simulink model "eFL_control"  (R2025b)
settings: Solver=ode3  StartTime=0.0  StopTime=1.5  FixedStep=1e-5  RelTol=1e-3  EnableMultiTasking=on
values from neighbouring files (symbols this model uses):
  C = 470*10^-6    (= 0.00047)    [plotting.m]    (also in robusnost_grafici.m)
  k0 = 2*200    (= 400)    [plotting.m]    (also in robusnost_grafici.m)
  k1 = 1    [plotting.m]    (also in robusnost_grafici.m)
  ki = 200^2    (= 40000)    [plotting.m]    (also in robusnost_grafici.m)
  L = 15.91*10^-3    (= 0.01591)    [plotting.m]    (also in robusnost_grafici.m = 0.012728)
  poremecaj = 0.8    [plotting.m]    (also in robusnost_grafici.m)
  R = 52    [plotting.m]    (also in robusnost_grafici.m)
  sig2 = (0.02*x2e)^2    (= 0.2025)    [plotting.m]    (also in robusnost_grafici.m = 0)
  x2e = Vc    (= -22.5)    [plotting.m]    (also in robusnost_grafici.m)
settings Model: Creator=Stevica  LastModifiedBy=User
settings SolverCC: AlgebraicLoopSolver=TrustRegion
settings DataIOCC: LimitDataPoints=on  SaveFormat=Array
settings OptimizationCC: LifeSpan=inf
settings DebuggingCC: UnderspecifiedInitializationDetection=Classic  MergeDetectMultiDrivingBlocksExec=none  SolverPrmCheckMsg=warning  UnconnectedInputMsg=warning  UnconnectedOutputMsg=warning  UnconnectedLineMsg=warning  SFUnexpectedBacktrackingDiag=warning  SFNoUnconditionalDefaultTransitionDiag=warning  SFExecutionAtInitializationDiag=none  ArithmeticOperatorsInVariantConditions=warning
settings HardwareCC: ProdBitPerPointer=32.0  ProdBitPerSizeT=32.0  ProdBitPerPtrDiffT=32.0  ProdLargestAtomicFloat=None  ProdIntDivRoundTo=Undefined  ProdEndianess=Unspecified  ProdWordSize=32.0  ProdHWDeviceType=32-bit Generic
settings ModelReferenceCC: PropagateSignalLabelsOutOfModel=off
settings SFSimCC: SimUseLocalCustomCode=off  CustomCodeUndefinedFunction=UseInterfaceOnly
settings RTWCC: RTWUseLocalCustomCode=off  GPUComputeCapability=3.5
settings CodeAppCC: StateflowObjectComments=on
settings GRTTargetCC: TargetLangStandard=C89/C90 (ANSI)
settings ConfigComp: CovMetricSettings=dw  CovSaveCumulativeToWorkspaceVar=on  CovSaveSingleToWorkspaceVar=on  CovExternalEMLEnable=off

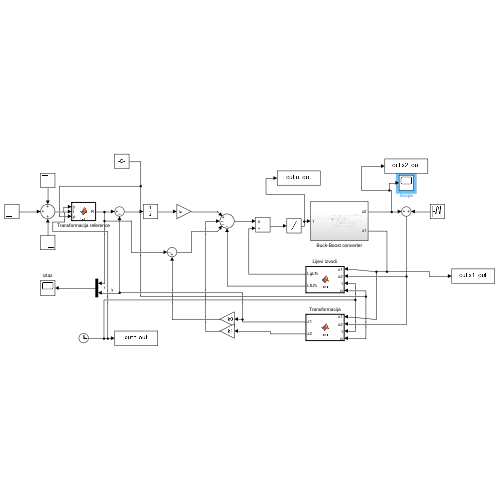
[thumbnail: Simulink's stored preview of the top-level diagram]
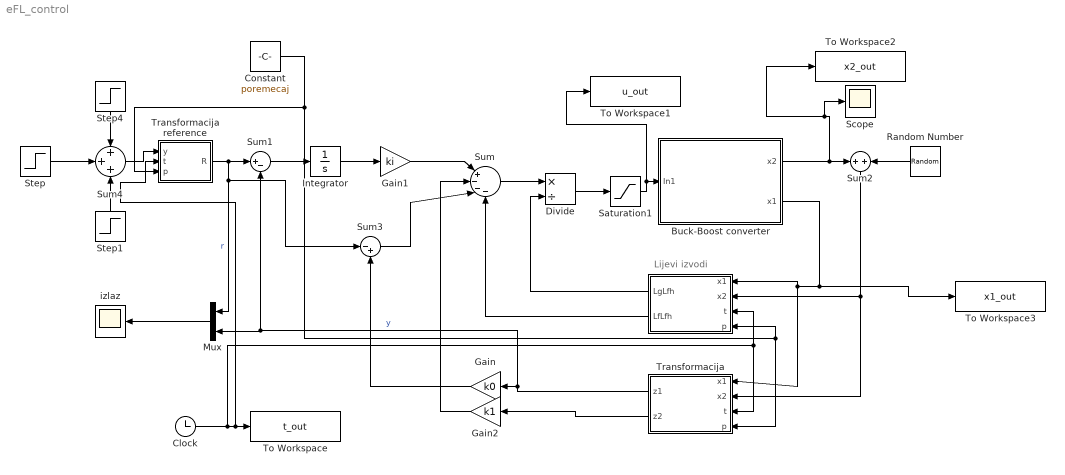
== system eFL_control ==
  note: Lijevi izvodi
  " " : MATLAB Function  TreatAsAtomicUnit=on
  Buck-Boost converter : Subsystem
  Clock : Clock
  Constant : Constant  Value=poremecaj
  Divide : Product  Inputs=*/
  Gain : Gain  Gain=k0
  Gain1 : Gain  Gain=ki
  Gain2 : Gain  Gain=k1
  Integrator : Integrator
  Mux : Mux  Inputs=2
  Random Number : RandomNumber  Variance=sig2  SampleTime=1e-5
  Saturation1 : Saturate  UpperLimit=1  LowerLimit=0
  Scope : Scope
      settings: ActiveDisplayYMinimum=-204.66780183595804  ActiveDisplayYMaximum=174.47139905299721
  Step : Step  Time=0.5  After=5  SampleTime=0
  Step1 : Step  After=-5  SampleTime=0
  Step4 : Step  Time=0  After=x2e  SampleTime=0
  Sum : Sum  Inputs=|+---
  Sum1 : Sum  Inputs=|+-
  Sum2 : Sum
  Sum3 : Sum  Inputs=|-+
  Sum4 : Sum  Inputs=+++
  To Workspace : ToWorkspace  VariableName=t_out  SampleTime=-1
  To Workspace1 : ToWorkspace  VariableName=u_out  SampleTime=-1
  To Workspace2 : ToWorkspace  VariableName=x2_out  SampleTime=-1
  To Workspace3 : ToWorkspace  VariableName=x1_out  SampleTime=-1
  Transformacija : MATLAB Function  TreatAsAtomicUnit=on
  Transformacija reference : MATLAB Function  TreatAsAtomicUnit=on
  izlaz : Scope
      settings: ActiveDisplayYMinimum=-0.63934283688742022  ActiveDisplayYMaximum=0.23107974343159757  DataLoggingVariableName=ScopeData2
  wires:
  " "/1(LgLfh) -> Divide/2
  Sum/1 -> Divide/1
  " "/2(LfLfh) -> Sum/4
  Transformacija/2(z2) -> Gain2/1
  Gain1/1 -> Sum/1
  Integrator/1 -> Gain1/1
  Gain2/1 -> Sum/2
  Divide/1 -> Saturation1/1
  Transformacija/1(z1) -> Mux/2, Sum1/2, Gain/1  "y"
  Mux/1 -> izlaz/1
  Sum1/1 -> Integrator/1
  Sum4/1 -> Transformacija reference/1(y)
  Transformacija reference/1(R) -> Sum3/1, Mux/1, Sum1/1  "r"
  Step/1 -> Sum4/2
  Step1/1 -> Sum4/3
  Step4/1 -> Sum4/1
  Saturation1/1 -> To Workspace1/1, Buck-Boost converter/1(In1)
  Random Number/1 -> Sum2/2
  Clock/1 -> To Workspace/1, Transformacija reference/2(t), Transformacija/3(t), " "/3(t)
  Buck-Boost converter/2(x1) -> To Workspace3/1, Transformacija/1(x1), " "/1(x1)
  Buck-Boost converter/1(x2) -> To Workspace2/1, Scope/1, Sum2/1
  Sum2/1 -> Transformacija/2(x2), " "/2(x2)
  Gain/1 -> Sum3/2
  Sum3/1 -> Sum/3
  Constant/1 -> Transformacija/4(p), " "/4(p), Transformacija reference/3(p)

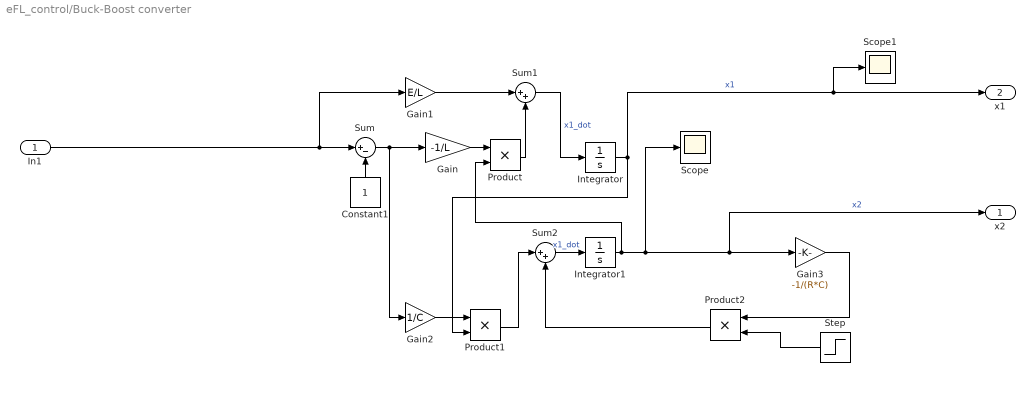
== system eFL_control/Buck-Boost converter ==
  In1 : Inport
  Constant1 : Constant
  Gain : Gain  Gain=-1/L
  Gain1 : Gain  Gain=E/L
  Gain2 : Gain  Gain=1/C
  Gain3 : Gain  Gain=-1/(R*C)
  Integrator : Integrator
  Integrator1 : Integrator
  Product : Product
  Product1 : Product
  Product2 : Product
  Scope : Scope
      settings: ActiveDisplayYMinimum=-124.96929112712884  ActiveDisplayYMaximum=85.0523446859199  DataLoggingVariableName=ScopeData8
  Scope1 : Scope
      settings: ActiveDisplayYMinimum=-26.319279231157857  ActiveDisplayYMaximum=-12.138137358974118  DataLoggingVariableName=ScopeData8
  Step : Step  Time=1.3  Before=1  After=1/poremecaj  SampleTime=0
  Sum : Sum  Inputs=|+-
  Sum1 : Sum  Inputs=|++
  Sum2 : Sum  Inputs=|++
  x2 : Outport
  x1 : Outport  Port=2
  wires:
  Gain/1 -> Product/1
  In1/1 -> Gain1/1, Sum/1
  Sum1/1 -> Integrator/1  "x1_dot"
  Gain1/1 -> Sum1/1
  Sum/1 -> Gain2/1, Gain/1
  Constant1/1 -> Sum/2
  Gain2/1 -> Product1/1
  Product/1 -> Sum1/2
  Integrator1/1 -> x2/1, Gain3/1, Scope/1, Product/2  "x2"
  Product1/1 -> Sum2/1
  Integrator/1 -> Scope1/1, x1/1, Product1/2  "x1"
  Sum2/1 -> Integrator1/1  "x1_dot"
  Gain3/1 -> Product2/1
  Product2/1 -> Sum2/2
  Step/1 -> Product2/2

== matlab function eFL_control/Transformacija ==
  data: x1 input; x2 input; z1 output; z2 output; t input; p input
function [z1, z2] = fcn(x1, x2,t, p)

L=15.91*10^-3;
C=470*10^-6;
if t < 1.3
    R = 52;
else
    R = 52*p;
end
E=12;

Vc=-22.5;
x2e=Vc;
x1e=1.2441;


z1 = C*x2^2 - 2*E*C*x2 + L*x1^2 + C*E^2 - (C*x2e^2 - 2*E*C*x2e + L*x1e^2 + C*E^2);
z2 = -2/R*x2^2 + 2*E*x1 + 2*E/R*x2;

== matlab function eFL_control/  ==
  data: x1 input; x2 input; LgLfh output; LfLfh output; t input; p input
function [LgLfh, LfLfh] = fcn(x1, x2,t, p)

L=15.91*10^-3;
C=470*10^-6;
if t < 1.3
    R = 52;
else
    R = 52*p;
end
E=12;

LgLfh = -4/(R*C)*x1*x2 + 2*E/(R*C)*x1 + 2*E^2/L - 2*E/L*x2;
LfLfh = 4/(R^2*C)*x2^2 - 2*E/(R^2*C)*x2 + 2*E/L*x2...
    - 2*E/(R*C)*x1 +4/(R*C)*x1*x2;

== matlab function eFL_control/Transformacija reference ==
  data: y input; R output; t input; p input
function  R= fcn(y,t, p)

L=15.91*10^-3;
C=470*10^-6;
if t < 1.3
    R = 52;
else
    R = 52*p;
end
E=12;

Vc=-22.5;
x2e=Vc;
x1e=1.2441;

gama = C*x2e^2 - 2*E*C*x2e + L*x1e^2;

R = C*y^2 - 2*E*C*y + L*(y*(y-E)/(R*E))^2 - gama;
